simulink model "Heating_room_quick"  (R2023b)
settings: Solver=VariableStepAuto  StartTime=0.0  StopTime=7000  RelTol=1e-3
libraries: fl_lib x21, SimscapeFluids_lib x4, nesl_utility x3
settings Model: Creator=Fahim  LastModifiedBy=Tanzi
settings SimscapeCC: SimscapeLogType=all

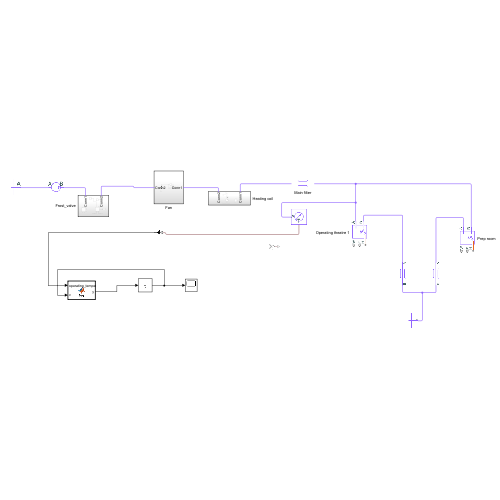
[thumbnail: Simulink's stored preview of the top-level diagram]
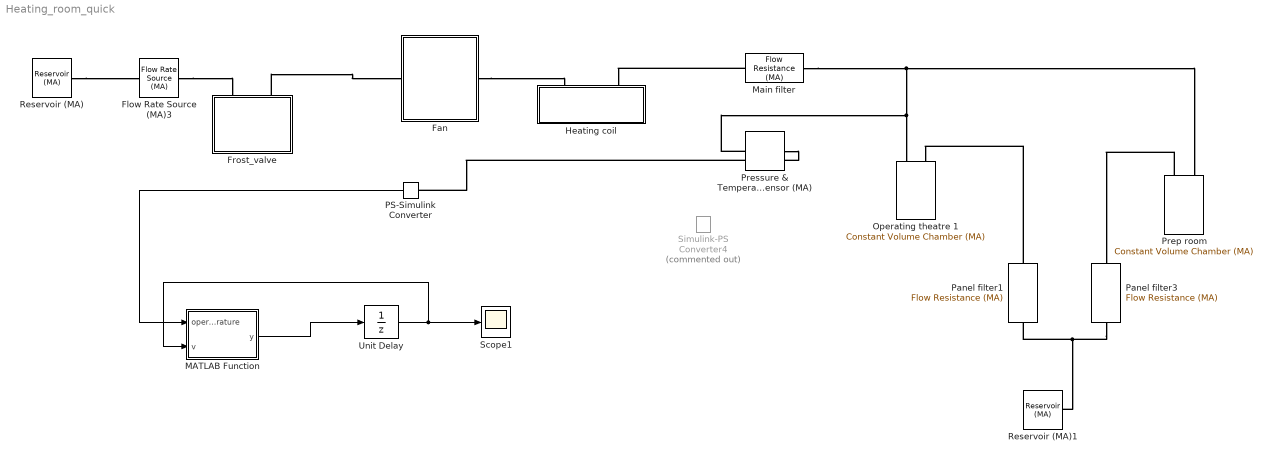
== system Heating_room_quick ==
  Fan : Subsystem
  Flow Rate Source (MA)3 : fl_lib/Moist Air/Sources/Flow Rate Source (MA)  source_type=foundation.enum.constant_controlled.constant  flow_type=foundation.enum.mass_volumetric_flow.mass  mass_flow=1.2 kg/s  volumetric_flow=1 m^3/s  volumetric_flow_conditions=foundation.enum.volumetric_flow_conditions.actual  p_std=0.101325 MPa  T_std=20 degC  RH_std=0.65  power_spec=foundation.enum.power_spec.none  area_A=1.2 m^2  area_B=1.2 m^2
      settings: InternalSimscapePortConfiguration="{\"Bottom\":[],\"Left\":[{\"id\":\"A\",\"label\":\"A\",\"type\":\"foundation.moist_air.moist_air\"}],\"Right\":[{\"id\":\"B\",\"label\":\"B\",\"type\":\"foundation.moist_air.moist_air\"}],\"Top\":[]}"
  Frost_valve : Subsystem
  Heating coil : Subsystem
  MATLAB Function : MATLAB Function  TreatAsAtomicUnit=on
  Main filter : fl_lib/Moist Air/Elements/Flow Resistance (MA)  delta_p_nominal=0.001 MPa  mdot_nominal=2.7 kg/s  rho_nominal=1.2 kg/m^3  area=1.2 m^2  laminar_fraction=1e-3
  Operating theatre 1 : fl_lib/Moist Air/Elements/Constant Volume Chamber (MA)  volume=157 m^3  num_ports=foundation.enum.num_ports.two  area_A=1.2 m^2  area_B=1.2 m^2  area_C=1.2 m^2  area_D=0.01 m^2  RH_ws=1  time_constant=1e-3 s  moisture_trace_gas_source=foundation.enum.moisture_trace_gas_source.none  moisture_source_spec=foundation.enum.moisture_source_spec.vapor  moisture_mass_flow=0 kg/s  moisture_temperature_spec=foundation.enum.temperature_spec.atmospheric  moisture_temperature=293.15 K  trace_gas_mass_flow=0 kg/s  trace_gas_temperature_spec=foundation.enum.temperature_spec.atmospheric  trace_gas_temperature=293.15 K  p_I_specify=off  p_I_priority=High  p_I=0.101325 MPa  p_I_nominal_specify=off  p_I_nominal_unit=MPa  p_I_nominal_value=1  T_I_specify=off  T_I_priority=High  T_I=293.15 K  T_I_nominal_specify=off  T_I_nominal_unit=K  T_I_nominal_value=1  RH_I_specify=off  RH_I_priority=High  RH_I=0  RH_I_nominal_specify=off  RH_I_nominal_unit=1  RH_I_nominal_value=1  x_w_I_specify=off  x_w_I_priority=None  x_w_I=0  x_w_I_nominal_specify=off  x_w_I_nominal_unit=1  x_w_I_nominal_value=1  y_w_I_specify=off  y_w_I_priority=None  y_w_I=0  y_w_I_nominal_specify=off  y_w_I_nominal_unit=1  y_w_I_nominal_value=1  HR_I_specify=off  HR_I_priority=None  HR_I=0  HR_I_nominal_specify=off  HR_I_nominal_unit=1  HR_I_nominal_value=1  x_g_I_specify=off  x_g_I_priority=High  x_g_I=0  x_g_I_nominal_specify=off  x_g_I_nominal_unit=1  x_g_I_nominal_value=1  y_g_I_specify=off  y_g_I_priority=None  y_g_I=0  y_g_I_nominal_specify=off  y_g_I_nominal_unit=1  y_g_I_nominal_value=1
      settings: InternalSimscapePortConfiguration="{\"Bottom\":[],\"Left\":[{\"id\":\"A\",\"label\":\"A\",\"type\":\"foundation.moist_air.moist_air\"},{\"id\":\"B\",\"label\":\"B\",\"type\":\"foundation.moist_air.moist_air\"}],\"Right\":[{\"id\":\"W\",\"label\":\"W\",\"type\":\"output\"},{\"id\":\"F\",\"label\":\"F\",\"type\":\"output\"},{\"id\":\"H\",\"label\":\"H\",\"type\":\"foundation.thermal.thermal\"}],\"Top\":[]}"
  PS-Simulink Converter : nesl_utility/PS-Simulink Converter  PhysicalDomain=network_engine_domain  SubClassName=ps_output  LeftPortType=input  RightPortType=output  PseudoPeriodic=off  Frequencies=[]  VectorFormat=inherit  Unit=inherit  AffineConversion=off
  Panel filter1 : fl_lib/Moist Air/Elements/Flow Resistance (MA)  delta_p_nominal=0.001 MPa  mdot_nominal=0.1 kg/s  rho_nominal=0 kg/m^3  area=0.01 m^2  laminar_fraction=1e-3
  Panel filter3 : fl_lib/Moist Air/Elements/Flow Resistance (MA)  delta_p_nominal=0.001 MPa  mdot_nominal=0.1 kg/s  rho_nominal=0 kg/m^3  area=0.01 m^2  laminar_fraction=1e-3
  Prep room : fl_lib/Moist Air/Elements/Constant Volume Chamber (MA)  volume=157 m^3  num_ports=foundation.enum.num_ports.two  area_A=1.2 m^2  area_B=1.2 m^2  area_C=1.2 m^2  area_D=0.01 m^2  RH_ws=1  time_constant=1e-3 s  moisture_trace_gas_source=foundation.enum.moisture_trace_gas_source.none  moisture_source_spec=foundation.enum.moisture_source_spec.vapor  moisture_mass_flow=0 kg/s  moisture_temperature_spec=foundation.enum.temperature_spec.atmospheric  moisture_temperature=293.15 K  trace_gas_mass_flow=0 kg/s  trace_gas_temperature_spec=foundation.enum.temperature_spec.atmospheric  trace_gas_temperature=293.15 K  p_I_specify=off  p_I_priority=High  p_I=0.101325 MPa  p_I_nominal_specify=off  p_I_nominal_unit=MPa  p_I_nominal_value=1  T_I_specify=off  T_I_priority=High  T_I=293.15 K  T_I_nominal_specify=off  T_I_nominal_unit=K  T_I_nominal_value=1  RH_I_specify=off  RH_I_priority=High  RH_I=0  RH_I_nominal_specify=off  RH_I_nominal_unit=1  RH_I_nominal_value=1  x_w_I_specify=off  x_w_I_priority=None  x_w_I=0  x_w_I_nominal_specify=off  x_w_I_nominal_unit=1  x_w_I_nominal_value=1  y_w_I_specify=off  y_w_I_priority=None  y_w_I=0  y_w_I_nominal_specify=off  y_w_I_nominal_unit=1  y_w_I_nominal_value=1  HR_I_specify=off  HR_I_priority=None  HR_I=0  HR_I_nominal_specify=off  HR_I_nominal_unit=1  HR_I_nominal_value=1  x_g_I_specify=off  x_g_I_priority=High  x_g_I=0  x_g_I_nominal_specify=off  x_g_I_nominal_unit=1  x_g_I_nominal_value=1  y_g_I_specify=off  y_g_I_priority=None  y_g_I=0  y_g_I_nominal_specify=off  y_g_I_nominal_unit=1  y_g_I_nominal_value=1
      settings: InternalSimscapePortConfiguration="{\"Bottom\":[],\"Left\":[{\"id\":\"A\",\"label\":\"A\",\"type\":\"foundation.moist_air.moist_air\"},{\"id\":\"B\",\"label\":\"B\",\"type\":\"foundation.moist_air.moist_air\"}],\"Right\":[{\"id\":\"W\",\"label\":\"W\",\"type\":\"output\"},{\"id\":\"F\",\"label\":\"F\",\"type\":\"output\"},{\"id\":\"H\",\"label\":\"H\",\"type\":\"foundation.thermal.thermal\"}],\"Top\":[]}"
  Pressure & Temperature Sensor (MA) : fl_lib/Moist Air/Sensors/Pressure & Temperature Sensor (MA)  reference=foundation.enum.MeasurementReference.absolute  pressure=false  pressure_spec=foundation.enum.PressureMeasementSpec.Absolute  temperature=true
      settings: InternalSimscapePortConfiguration="{\"Bottom\":[{\"id\":\"T\",\"label\":\"T\",\"type\":\"output\"}],\"Left\":[{\"id\":\"A\",\"label\":\"A\",\"type\":\"foundation.moist_air.moist_air\"}],\"Right\":[],\"Top\":[]}"
  Reservoir (MA) : fl_lib/Moist Air/Elements/Reservoir (MA)  pressure_spec=foundation.enum.pressure_spec.atmospheric  reservoir_pressure=0.101325 MPa  temperature_spec=foundation.enum.temperature_spec.specified  reservoir_temperature=8 degC  moisture_spec=foundation.enum.moistureSpec.RelativeHumidity  reservoir_RH=0.5  reservoir_x_w=0.01  reservoir_y_w=0.01  reservoir_HR=0.01  reservoir_Tw=287 K  trace_gas_spec=foundation.enum.trace_gas_spec.mass_fraction  reservoir_x_g=0.001  reservoir_y_g=0.001  RH_ws=1  area_A=1.2 m^2
  Reservoir (MA)1 : fl_lib/Moist Air/Elements/Reservoir (MA)  pressure_spec=foundation.enum.pressure_spec.atmospheric  reservoir_pressure=0.101325 MPa  temperature_spec=foundation.enum.temperature_spec.specified  reservoir_temperature=18.5 degC  moisture_spec=foundation.enum.moistureSpec.RelativeHumidity  reservoir_RH=0.5  reservoir_x_w=0.01  reservoir_y_w=0.01  reservoir_HR=0.01  reservoir_Tw=287 K  trace_gas_spec=foundation.enum.trace_gas_spec.mass_fraction  reservoir_x_g=0.001  reservoir_y_g=0.001  RH_ws=1  area_A=1.2 m^2
  Scope1 : Scope
  Simulink-PS Converter4 : nesl_utility/Simulink-PS Converter  Commented=on  PhysicalDomain=network_engine_domain  SubClassName=ps_input  LeftPortType=input  RightPortType=output  PseudoPeriodic=off  Frequencies=[]  NoiseDistribution=none  NoiseParameters=[]  Unit=1  AffineConversion=off  FilteringAndDerivatives=provide  SimscapeFilterOrder=1  InputFilterTimeConstant=0.001  UdotUserProvided=0
  Unit Delay : UnitDelay  InitialCondition=8+273  SampleTime=-1  StateName=current_temp  HasFrameUpgradeWarning=on
  wires:
  PS-Simulink Converter/1 -> MATLAB Function/1(operating_temperature)
  MATLAB Function/1(y) -> Unit Delay/1
  Unit Delay/1 -> MATLAB Function/2(v), Scope1/1
  connections:
  Reservoir (MA)/LConn1 -- Flow Rate Source (MA)3/LConn1
  Flow Rate Source (MA)3/RConn1 -- Frost_valve/RConn1
  Frost_valve/RConn2 -- Fan/LConn1
  Fan/RConn1 -- Heating coil/RConn1
  Main filter/LConn1 -- Heating coil/RConn2
  Panel filter3/RConn1 -- Panel filter1/RConn1 -- Reservoir (MA)1/LConn1
  Prep room/LConn1 -- Panel filter3/LConn1
  Panel filter1/LConn1 -- Operating theatre 1/LConn2
  Main filter/RConn1 -- Pressure & Temperature Sensor (MA)/LConn1 -- Operating theatre 1/LConn1 -- Prep room/LConn2
  Pressure & Temperature Sensor (MA)/RConn1 -- PS-Simulink Converter/LConn1

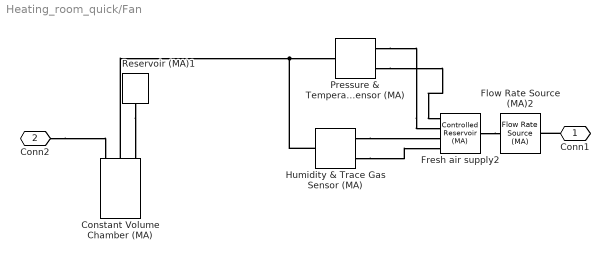
== system Heating_room_quick/Fan ==
  Constant Volume Chamber (MA) : fl_lib/Moist Air/Elements/Constant Volume Chamber (MA)  volume=3.6 m^3  num_ports=foundation.enum.num_ports.three  area_A=1.2 m^2  area_B=1.2 m^2  area_C=1.2 m^2  area_D=0.01 m^2  RH_ws=1  time_constant=1e-3 s  moisture_trace_gas_source=foundation.enum.moisture_trace_gas_source.none  moisture_source_spec=foundation.enum.moisture_source_spec.vapor  moisture_mass_flow=0 kg/s  moisture_temperature_spec=foundation.enum.temperature_spec.atmospheric  moisture_temperature=293.15 K  trace_gas_mass_flow=0 kg/s  trace_gas_temperature_spec=foundation.enum.temperature_spec.atmospheric  trace_gas_temperature=293.15 K  p_I_specify=off  p_I_priority=High  p_I=0.101325 MPa  p_I_nominal_specify=off  p_I_nominal_unit=MPa  p_I_nominal_value=1  T_I_specify=off  T_I_priority=High  T_I=293.15 K  T_I_nominal_specify=off  T_I_nominal_unit=K  T_I_nominal_value=1  RH_I_specify=off  RH_I_priority=High  RH_I=0  RH_I_nominal_specify=off  RH_I_nominal_unit=1  RH_I_nominal_value=1  x_w_I_specify=off  x_w_I_priority=None  x_w_I=0  x_w_I_nominal_specify=off  x_w_I_nominal_unit=1  x_w_I_nominal_value=1  y_w_I_specify=off  y_w_I_priority=None  y_w_I=0  y_w_I_nominal_specify=off  y_w_I_nominal_unit=1  y_w_I_nominal_value=1  HR_I_specify=off  HR_I_priority=None  HR_I=0  HR_I_nominal_specify=off  HR_I_nominal_unit=1  HR_I_nominal_value=1  x_g_I_specify=off  x_g_I_priority=High  x_g_I=0  x_g_I_nominal_specify=off  x_g_I_nominal_unit=1  x_g_I_nominal_value=1  y_g_I_specify=off  y_g_I_priority=None  y_g_I=0  y_g_I_nominal_specify=off  y_g_I_nominal_unit=1  y_g_I_nominal_value=1
      settings: InternalSimscapePortConfiguration="{\"Bottom\":[],\"Left\":[{\"id\":\"A\",\"label\":\"A\",\"type\":\"foundation.moist_air.moist_air\"},{\"id\":\"B\",\"label\":\"B\",\"type\":\"foundation.moist_air.moist_air\"},{\"id\":\"C\",\"label\":\"C\",\"type\":\"foundation.moist_air.moist_air\"}],\"Right\":[{\"id\":\"W\",\"label\":\"W\",\"type\":\"output\"},{\"id\":\"F\",\"label\":\"F\",\"type\":\"output\"},{\"id\":\"H\",\"label\":\"H\",\"type\":\"foundation.thermal.thermal\"}],\"Top\":[]}"
  Flow Rate Source (MA)2 : fl_lib/Moist Air/Sources/Flow Rate Source (MA)  source_type=foundation.enum.constant_controlled.constant  flow_type=foundation.enum.mass_volumetric_flow.mass  mass_flow=2.7 kg/s  volumetric_flow=1 m^3/s  volumetric_flow_conditions=foundation.enum.volumetric_flow_conditions.actual  p_std=0.101325 MPa  T_std=20 degC  RH_std=0.65  power_spec=foundation.enum.power_spec.none  area_A=1.2 m^2  area_B=1.2 m^2
      settings: InternalSimscapePortConfiguration="{\"Bottom\":[],\"Left\":[{\"id\":\"A\",\"label\":\"A\",\"type\":\"foundation.moist_air.moist_air\"}],\"Right\":[{\"id\":\"B\",\"label\":\"B\",\"type\":\"foundation.moist_air.moist_air\"}],\"Top\":[]}"
  Fresh air supply2 : fl_lib/Moist Air/Elements/Controlled Reservoir (MA)  moisture_spec=foundation.enum.moistureSpec.RelativeHumidity  trace_gas_spec=foundation.enum.trace_gas_spec.mass_fraction  RH_ws=1  area_A=1.2 m^2  input_error_spec=foundation.enum.input_range_error.error
      settings: InternalSimscapePortConfiguration="{\"Bottom\":[],\"Left\":[{\"id\":\"A\",\"label\":\"A\",\"type\":\"foundation.moist_air.moist_air\"}],\"Right\":[{\"id\":\"T\",\"label\":\"T\",\"type\":\"input\"},{\"id\":\"P\",\"label\":\"P\",\"type\":\"input\"},{\"id\":\"W\",\"label\":\"W\",\"type\":\"input\"},{\"id\":\"G\",\"label\":\"G\",\"type\":\"input\"}],\"Top\":[]}"
  Humidity & Trace Gas Sensor (MA) : fl_lib/Moist Air/Sensors/Humidity & Trace Gas Sensor (MA)  moisture_on=true  moisture_spec=foundation.enum.moistureSpec.RelativeHumidity  trace_gas_on=true  trace_gas_spec=foundation.enum.trace_gas_spec.mass_fraction
      settings: InternalSimscapePortConfiguration="{\"Bottom\":[],\"Left\":[{\"id\":\"A\",\"label\":\"A\",\"type\":\"foundation.moist_air.moist_air\"}],\"Right\":[{\"id\":\"W\",\"label\":\"W\",\"type\":\"output\"},{\"id\":\"G\",\"label\":\"G\",\"type\":\"output\"}],\"Top\":[]}"
  Pressure & Temperature Sensor (MA) : fl_lib/Moist Air/Sensors/Pressure & Temperature Sensor (MA)  reference=foundation.enum.MeasurementReference.absolute  pressure=true  pressure_spec=foundation.enum.PressureMeasementSpec.Absolute  temperature=true
      settings: InternalSimscapePortConfiguration="{\"Bottom\":[{\"id\":\"T\",\"label\":\"T\",\"type\":\"output\"}],\"Left\":[{\"id\":\"A\",\"label\":\"A\",\"type\":\"foundation.moist_air.moist_air\"}],\"Right\":[{\"id\":\"Pa\",\"label\":\"Pa\",\"type\":\"output\"}],\"Top\":[]}"
  Reservoir (MA)1 : fl_lib/Moist Air/Elements/Reservoir (MA)  pressure_spec=foundation.enum.pressure_spec.atmospheric  reservoir_pressure=0.101325 MPa  temperature_spec=foundation.enum.temperature_spec.specified  reservoir_temperature=20 degC  moisture_spec=foundation.enum.moistureSpec.RelativeHumidity  reservoir_RH=0.5  reservoir_x_w=0.01  reservoir_y_w=0.01  reservoir_HR=0.01  reservoir_Tw=287 K  trace_gas_spec=foundation.enum.trace_gas_spec.mass_fraction  reservoir_x_g=0.001  reservoir_y_g=0.001  RH_ws=1  area_A=1.2 m^2
  Conn1 : PMIOPort  Side=Right
  Conn2 : PMIOPort  Port=2  Side=Left
  connections:
  Humidity & Trace Gas Sensor (MA)/RConn2 -- Fresh air supply2/RConn4
  Pressure & Temperature Sensor (MA)/RConn2 -- Fresh air supply2/RConn1
  Fresh air supply2/LConn1 -- Flow Rate Source (MA)2/LConn1
  Conn1/RConn1 -- Flow Rate Source (MA)2/RConn1
  Reservoir (MA)1/LConn1 -- Constant Volume Chamber (MA)/LConn3
  Humidity & Trace Gas Sensor (MA)/LConn1 -- Constant Volume Chamber (MA)/LConn2 -- Pressure & Temperature Sensor (MA)/LConn1
  Pressure & Temperature Sensor (MA)/RConn1 -- Fresh air supply2/RConn2
  Humidity & Trace Gas Sensor (MA)/RConn1 -- Fresh air supply2/RConn3
  Conn2/RConn1 -- Constant Volume Chamber (MA)/LConn1

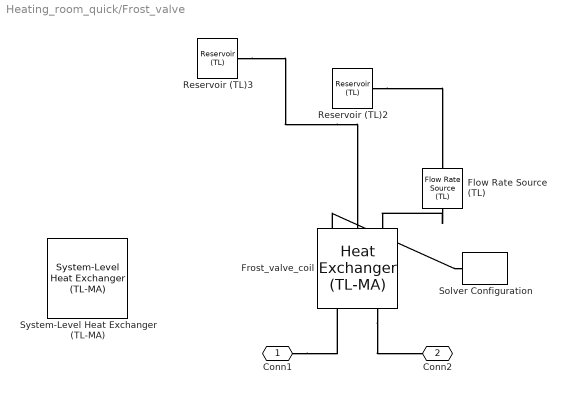
== system Heating_room_quick/Frost_valve ==
  Flow Rate Source (TL) : fl_lib/Thermal Liquid/Sources/Flow Rate Source (TL)  source_type=foundation.enum.constant_controlled.constant  flow_type=foundation.enum.mass_volumetric_flow.mass  mass_flow=0.31 kg/s  volumetric_flow=0 m^3/s  power_spec=foundation.enum.power_spec.none  area=0.44 in^2
      settings: InternalSimscapePortConfiguration="{\"Bottom\":[],\"Left\":[{\"id\":\"A\",\"label\":\"A\",\"type\":\"foundation.thermal_liquid.thermal_liquid\"}],\"Right\":[{\"id\":\"B\",\"label\":\"B\",\"type\":\"foundation.thermal_liquid.thermal_liquid\"}],\"Top\":[]}"
  Frost_valve_coil : SimscapeFluids_lib/Fluid Network Interfaces/Heat Exchangers/Heat Exchanger (TL-MA)  flow_arrangement=fluids.interfaces.heat_exchangers.enum.FlowArrangementTLMA.Cross  cross_flow_arrangement=fluids.interfaces.heat_exchangers.enum.CrossFlowArrangementTLMA.UnmixedUnmixed  R_wall=0 K/kW  area_A1=0.44 in^2  area_B1=0.44 in^2  area_A2=1.2 m^2  area_B2=1.2 m^2  flow_geometry_TL=fluids.interfaces.heat_exchangers.enum.FlowGeometryTL.InsideTubes  tube_num_TL=14  tube_length_TL=1.2 m  tube_cross_section_TL=fluids.interfaces.heat_exchangers.enum.TubeCrossSection.Circular  tube_diameter_TL=0.55 in  tube_width_TL=0.05 m  tube_height_TL=0.05 m  tube_inner_diameter_TL=0.05 m  tube_outer_diameter_TL=0.1 m  tube_flow_area_TL=0.002 m^2  tube_wetted_perimeter_TL=0.15 m  tube_heat_perimeter_TL=0.15 m  tube_pressure_loss_spec_TL=fluids.interfaces.heat_exchangers.enum.TubePressureLossSpec.Haaland  tube_loss_coeff_TL=10  tube_local_pressure_loss_spec_TL=fluids.thermal_liquid.pipes_fittings.enum.LocalLossSpec.AggregateLength  tube_length_add_TL=0.024 in  tube_local_loss_coefficient_TL=0.1  tube_roughness_pressure_TL=15e-6 m  tube_Re_lam_pressure_TL=2000  tube_Re_tur_pressure_TL=4000  tube_shape_factor_generic_TL=64  tube_heat_coeff_spec_TL=fluids.interfaces.heat_exchangers.enum.TubeHeatCoeffSpec.Gneilinski  tube_colburn_coeff_TL=[.023, .8, .33]  tube_roughness_heat_TL=15e-6 m  tube_Re_lam_heat_TL=2000  tube_Re_tur_heat_TL=4000  tube_Nu_lam_generic_TL=3.66  bank_arrangement_TL=fluids.interfaces.heat_exchangers.enum.BankArrangement.Inline  bank_num_rows_TL=5  bank_tubes_per_row_TL=5  bank_width_TL=1 m  bank_tube_diameter_TL=0.05 m  bank_longitudinal_pitch_TL=0.15 m  bank_transverse_pitch_TL=0.15 m  bank_pressure_loss_spec_TL=fluids.interfaces.heat_exchangers.enum.BankPressureLossSpec.Martin  bank_euler_TL=10  bank_heat_coeff_spec_TL=fluids.interfaces.heat_exchangers.enum.BankHeatCoeffSpec.Martin  bank_colburn_coeff_TL=[.27, .63, .36]  generic_flow_area_TL=0.01 m^2  generic_heat_area_TL=2 m^2  generic_volume_TL=0.05 m^3  generic_loss_coeff_TL=10  generic_colburn_coeff_TL=[.023, .8, .33]  fouling_factor_TL=0 K*m^2/kW  fin_area_TL=0 mm^2  fin_efficiency_TL=0.5  p_init_TL=1 bar  T_init_TL=99 degC  flow_geometry_MA=fluids.interfaces.heat_exchangers.enum.FlowGeometryMA.AcrossTubeBank  tube_num_MA=25  tube_length_MA=1 m  tube_cross_section_MA=fluids.interfaces.heat_exchangers.enum.TubeCrossSection.Circular  tube_diameter_MA=0.05 m  tube_width_MA=0.05 m  tube_height_MA=0.05 m  tube_inner_diameter_MA=0.05 m  tube_outer_diameter_MA=0.1 m  tube_flow_area_MA=0.002 m^2  tube_wetted_perimeter_MA=0.15 m  tube_heat_perimeter_MA=0.15 m  tube_pressure_loss_spec_MA=fluids.interfaces.heat_exchangers.enum.TubePressureLossSpec.Haaland  tube_loss_coeff_MA=10  tube_local_pressure_loss_spec_MA=fluids.moist_air.pipes_fittings.enum.LocalLossSpec.AggregateLength  tube_length_add_MA=0.1 m  tube_local_loss_coefficient_MA=0.1  tube_roughness_pressure_MA=15e-6 m  tube_Re_lam_pressure_MA=2000  tube_Re_tur_pressure_MA=4000  tube_shape_factor_generic_MA=64  tube_heat_coeff_spec_MA=fluids.interfaces.heat_exchangers.enum.TubeHeatCoeffSpec.Gneilinski  tube_colburn_coeff_MA=[.023, .8, .33]  tube_roughness_heat_MA=15e-6 m  tube_Re_lam_heat_MA=2000  tube_Re_tur_heat_MA=4000  tube_Nu_lam_generic_MA=3.66  bank_arrangement_MA=fluids.interfaces.heat_exchangers.enum.BankArrangement.Inline  bank_num_rows_MA=1  bank_tubes_per_row_MA=14  bank_width_MA=1.2 m  bank_tube_diameter_MA=0.65 in  bank_longitudinal_pitch_MA=1.1 in  bank_transverse_pitch_MA=1.1 in  bank_pressure_loss_spec_MA=fluids.interfaces.heat_exchangers.enum.BankPressureLossSpec.Martin  bank_euler_MA=10  bank_heat_coeff_spec_MA=fluids.interfaces.heat_exchangers.enum.BankHeatCoeffSpec.Martin  bank_colburn_coeff_MA=[.27, .63, .36]  generic_flow_area_MA=288 in^2  generic_heat_area_MA=0.0511 m^2  generic_volume_MA=1728 in^3  generic_loss_coeff_MA=10  generic_colburn_coeff_MA=[.023, .8, .33]  fouling_factor_MA=0.1 K*m^2/kW  fin_area_MA=2000 in^2  fin_efficiency_MA=0.6  p_init_MA=1 atm  T_init_MA=14 degC  moisture_spec_MA=foundation.enum.moisture_spec.relative_humidity  RH_init_MA=0.8  x_w_init_MA=0.01  y_w_init_MA=0.01  HR_init_MA=0.01  trace_gas_spec_MA=foundation.enum.trace_gas_spec.mass_fraction  x_g_init_MA=0.001  y_g_init_MA=0.001  RH_ws_MA=1
      settings: InternalSimscapePortConfiguration="{\"Bottom\":[],\"Left\":[{\"id\":\"A1\",\"label\":\"A1\",\"type\":\"foundation.thermal_liquid.thermal_liquid\"},{\"id\":\"B1\",\"label\":\"B1\",\"type\":\"foundation.thermal_liquid.thermal_liquid\"}],\"Right\":[{\"id\":\"A2\",\"label\":\"A2\",\"type\":\"foundation.moist_air.moist_air\"},{\"id\":\"B2\",\"label\":\"B2\",\"type\":\"foundation.moist_air.moist_air\"}],\"Top\":[{\"id\":\"W\",\"label\":\"W\",\"type\":\"output\"}]}"
  Reservoir (TL)2 : fl_lib/Thermal Liquid/Elements/Reservoir (TL)  pressure_spec=foundation.enum.pressure_spec.specified  reservoir_pressure=1 bar  reservoir_temperature=99 degC  area=0.44 in^2
  Reservoir (TL)3 : fl_lib/Thermal Liquid/Elements/Reservoir (TL)  pressure_spec=foundation.enum.pressure_spec.specified  reservoir_pressure=1 bar  reservoir_temperature=89 degC  area=0.44 in^2
  Solver Configuration : nesl_utility/Solver Configuration  PhysicalDomain=network_engine_domain  SubClassName=solver  LeftPortType=input  RightPortType=generic  Tones=[]  Harmonics=[]  SimulateNoise=off  Profile=off  UseLocalSampling=off  EnableSwitchedLinearOptims=on  FrequencyDomain=off  UseCCode=off  RelTol=0.001  AbsTol=0.001  MinStep=1e-09  ToWorkspace=off  RevertToSquareIcSolve=off  NumHomotopyIterations=100  PhasorMode=off  PhasorModeNumHarmonics=1  ConsistencySolver=NEWTON_XTOL_AFTER_FTOL  IndexReductionMethod=DerivativeReplacement  DoDC=off  ResidualTolerance=1e-09  ConsistencyTolSource=GLOBAL  ConsistencyAbsTol=0.001  ConsistencyRelTol=0.001  ConsistencyTolFactor=0.001  UseLocalSolver=off  LocalSolverChoice=NE_BACKWARD_EULER_ADVANCER  ResolveIndetEquations=on  FunctionEvalNumThread=1  LocalSolverSampleTime=0.001  DoFixedCost=off  MaxNonlinIter=3  MaxModeIter=2  ComputeImpulses=off  ImpulseIterations=2  LinearAlgebra=auto  LinearAlgebraNumThread=0  EquationFormulation=NE_TIME_EF  DelaysMemoryBudget=1024  AutomaticFiltering=on  FilteringTimeConstant=0.001  PartitionStorageMethod=AS_NEEDED  PartitionMemoryBudget=1024  PartitionMethod=ROBUST  MultibodyUseLocalSolver=off  MultibodyLocalSolverChoice=ODE1  MultibodyLocalSolverSampleTime=0.001
  System-Level Heat Exchanger (TL-MA) : SimscapeFluids_lib/Fluid Network Interfaces/Heat Exchangers/System-Level Heat Exchanger (TL-MA)  flow_arrangement=fluids.interfaces.heat_exchangers.enum.SystemLevelFlowArrangementTLMA.Cross  wall_thermal_mass=false  mass_wall=1 kg  cp_wall=490 J/(K*kg)  nominal_init_wall=true  T_wall_init=293.15 K  area_A1=0.44 in^2  area_B1=0.44 in^2  area_A2=1.2 m^2  area_B2=1.2 m^2  operating_condition_TL=fluids.interfaces.heat_exchangers.enum.SystemLevelOperatingConditionTLMA.Cooling  mdot_nominal_TL=0.31 kg/s  delta_p_nominal_TL=8 kPa  p_in_nominal_TL=0.101325 MPa  T_in_nominal_TL=99 degC  capacity_spec_TL=fluids.interfaces.heat_exchangers.enum.SystemLevelCapacitySpec.HeatTransfer  Q_nominal=7 kW  T_out_nominal_TL=69 degC  volume_TL=0.00477 m^3  nominal_init_TL=true  p_init_TL=0.101325 MPa  T_init_TL=293.15 K  mdot_nominal_MA=1.2 kg/s  delta_p_nominal_MA=0.001 MPa  p_in_nominal_MA=0.101325 MPa  T_in_nominal_MA=10 degC  inlet_moisture_spec_MA=foundation.enum.moisture_spec.relative_humidity  RH_in_nominal_MA=0.5  x_w_in_nominal_MA=0.01  y_w_in_nominal_MA=0.01  HR_in_nominal_MA=0.01  inlet_trace_gas_spec_MA=foundation.enum.trace_gas_spec.mass_fraction  x_g_in_nominal_MA=0.001  y_g_in_nominal_MA=0.001  volume_MA=0.8 m^3  nominal_init_MA=true  p_init_MA=0.101325 MPa  T_init_MA=293.15 K  moisture_spec_MA=foundation.enum.moisture_spec.relative_humidity  RH_init_MA=0.5  x_w_init_MA=0.01  y_w_init_MA=0.01  HR_init_MA=0.01  trace_gas_spec_MA=foundation.enum.trace_gas_spec.mass_fraction  x_g_init_MA=0.001  y_g_init_MA=0.001  RH_ws_MA=1  a_TL=0.023  b_TL=0.8  c_TL=0.33  a_MA=0.023  b_MA=0.8  c_MA=0.33
      settings: InternalSimscapePortConfiguration="{\"Bottom\":[],\"Left\":[{\"id\":\"A1\",\"label\":\"A1\",\"type\":\"foundation.thermal_liquid.thermal_liquid\"},{\"id\":\"B1\",\"label\":\"B1\",\"type\":\"foundation.thermal_liquid.thermal_liquid\"}],\"Right\":[{\"id\":\"A2\",\"label\":\"A2\",\"type\":\"foundation.moist_air.moist_air\"},{\"id\":\"B2\",\"label\":\"B2\",\"type\":\"foundation.moist_air.moist_air\"}],\"Top\":[{\"id\":\"Q1\",\"label\":\"Q1\",\"type\":\"output\"},{\"id\":\"Q2\",\"label\":\"Q2\",\"type\":\"output\"},{\"id\":\"W\",\"label\":\"W\",\"type\":\"output\"}]}"
  Conn1 : PMIOPort  Side=Right
  Conn2 : PMIOPort  Port=2  Side=Right
  connections:
  Reservoir (TL)2/LConn1 -- Flow Rate Source (TL)/LConn1
  Flow Rate Source (TL)/RConn1 -- Frost_valve_coil/LConn1
  Reservoir (TL)3/LConn1 -- Frost_valve_coil/LConn2
  Conn1/RConn1 -- Frost_valve_coil/RConn2
  Frost_valve_coil/RConn1 -- Conn2/RConn1
  Frost_valve_coil/LConn3 -- Solver Configuration/RConn1

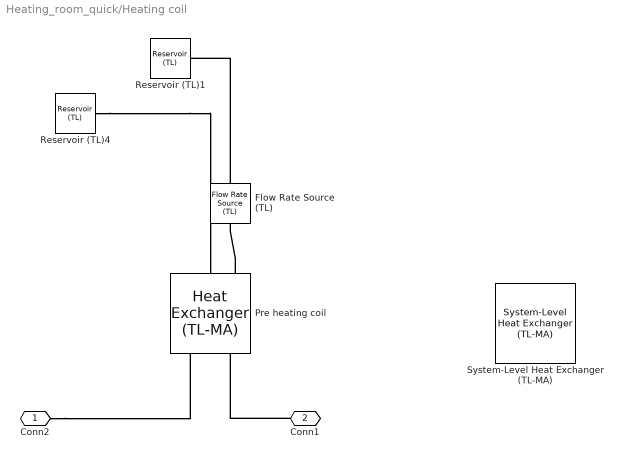
== system Heating_room_quick/Heating coil ==
  Flow Rate Source (TL) : fl_lib/Thermal Liquid/Sources/Flow Rate Source (TL)  source_type=foundation.enum.constant_controlled.constant  flow_type=foundation.enum.mass_volumetric_flow.mass  mass_flow=0.41 kg/s  volumetric_flow=0 m^3/s  power_spec=foundation.enum.power_spec.none  area=0.44 in^2
      settings: InternalSimscapePortConfiguration="{\"Bottom\":[],\"Left\":[{\"id\":\"A\",\"label\":\"A\",\"type\":\"foundation.thermal_liquid.thermal_liquid\"}],\"Right\":[{\"id\":\"B\",\"label\":\"B\",\"type\":\"foundation.thermal_liquid.thermal_liquid\"}],\"Top\":[]}"
  Pre heating coil : SimscapeFluids_lib/Fluid Network Interfaces/Heat Exchangers/Heat Exchanger (TL-MA)  flow_arrangement=fluids.interfaces.heat_exchangers.enum.FlowArrangementTLMA.Cross  cross_flow_arrangement=fluids.interfaces.heat_exchangers.enum.CrossFlowArrangementTLMA.UnmixedUnmixed  R_wall=0 K/kW  area_A1=0.44 in^2  area_B1=0.44 in^2  area_A2=1.2 m^2  area_B2=1.2 m^2  flow_geometry_TL=fluids.interfaces.heat_exchangers.enum.FlowGeometryTL.InsideTubes  tube_num_TL=14  tube_length_TL=1.2 m  tube_cross_section_TL=fluids.interfaces.heat_exchangers.enum.TubeCrossSection.Circular  tube_diameter_TL=0.55 in  tube_width_TL=0.05 m  tube_height_TL=0.05 m  tube_inner_diameter_TL=0.05 m  tube_outer_diameter_TL=0.1 m  tube_flow_area_TL=0.002 m^2  tube_wetted_perimeter_TL=0.15 m  tube_heat_perimeter_TL=0.15 m  tube_pressure_loss_spec_TL=fluids.interfaces.heat_exchangers.enum.TubePressureLossSpec.Haaland  tube_loss_coeff_TL=10  tube_local_pressure_loss_spec_TL=fluids.thermal_liquid.pipes_fittings.enum.LocalLossSpec.AggregateLength  tube_length_add_TL=0.024 in  tube_local_loss_coefficient_TL=0.1  tube_roughness_pressure_TL=15e-6 m  tube_Re_lam_pressure_TL=2000  tube_Re_tur_pressure_TL=4000  tube_shape_factor_generic_TL=64  tube_heat_coeff_spec_TL=fluids.interfaces.heat_exchangers.enum.TubeHeatCoeffSpec.Gneilinski  tube_colburn_coeff_TL=[.023, .8, .33]  tube_roughness_heat_TL=15e-6 m  tube_Re_lam_heat_TL=2000  tube_Re_tur_heat_TL=4000  tube_Nu_lam_generic_TL=3.66  bank_arrangement_TL=fluids.interfaces.heat_exchangers.enum.BankArrangement.Inline  bank_num_rows_TL=5  bank_tubes_per_row_TL=5  bank_width_TL=1 m  bank_tube_diameter_TL=0.05 m  bank_longitudinal_pitch_TL=0.15 m  bank_transverse_pitch_TL=0.15 m  bank_pressure_loss_spec_TL=fluids.interfaces.heat_exchangers.enum.BankPressureLossSpec.Martin  bank_euler_TL=10  bank_heat_coeff_spec_TL=fluids.interfaces.heat_exchangers.enum.BankHeatCoeffSpec.Martin  bank_colburn_coeff_TL=[.27, .63, .36]  generic_flow_area_TL=0.01 m^2  generic_heat_area_TL=2 m^2  generic_volume_TL=0.05 m^3  generic_loss_coeff_TL=10  generic_colburn_coeff_TL=[.023, .8, .33]  fouling_factor_TL=0 K*m^2/kW  fin_area_TL=0 mm^2  fin_efficiency_TL=0.5  p_init_TL=1 bar  T_init_TL=90 degC  flow_geometry_MA=fluids.interfaces.heat_exchangers.enum.FlowGeometryMA.AcrossTubeBank  tube_num_MA=25  tube_length_MA=1 m  tube_cross_section_MA=fluids.interfaces.heat_exchangers.enum.TubeCrossSection.Circular  tube_diameter_MA=0.05 m  tube_width_MA=0.05 m  tube_height_MA=0.05 m  tube_inner_diameter_MA=0.05 m  tube_outer_diameter_MA=0.1 m  tube_flow_area_MA=0.002 m^2  tube_wetted_perimeter_MA=0.15 m  tube_heat_perimeter_MA=0.15 m  tube_pressure_loss_spec_MA=fluids.interfaces.heat_exchangers.enum.TubePressureLossSpec.Haaland  tube_loss_coeff_MA=10  tube_local_pressure_loss_spec_MA=fluids.moist_air.pipes_fittings.enum.LocalLossSpec.AggregateLength  tube_length_add_MA=0.1 m  tube_local_loss_coefficient_MA=0.1  tube_roughness_pressure_MA=15e-6 m  tube_Re_lam_pressure_MA=2000  tube_Re_tur_pressure_MA=4000  tube_shape_factor_generic_MA=64  tube_heat_coeff_spec_MA=fluids.interfaces.heat_exchangers.enum.TubeHeatCoeffSpec.Gneilinski  tube_colburn_coeff_MA=[.023, .8, .33]  tube_roughness_heat_MA=15e-6 m  tube_Re_lam_heat_MA=2000  tube_Re_tur_heat_MA=4000  tube_Nu_lam_generic_MA=3.66  bank_arrangement_MA=fluids.interfaces.heat_exchangers.enum.BankArrangement.Inline  bank_num_rows_MA=1  bank_tubes_per_row_MA=14  bank_width_MA=1.2 m  bank_tube_diameter_MA=0.55 in  bank_longitudinal_pitch_MA=1.1 in  bank_transverse_pitch_MA=1.1 in  bank_pressure_loss_spec_MA=fluids.interfaces.heat_exchangers.enum.BankPressureLossSpec.Martin  bank_euler_MA=10  bank_heat_coeff_spec_MA=fluids.interfaces.heat_exchangers.enum.BankHeatCoeffSpec.Martin  bank_colburn_coeff_MA=[.27, .63, .36]  generic_flow_area_MA=288 in^2  generic_heat_area_MA=0.0511 m^2  generic_volume_MA=1728 in^3  generic_loss_coeff_MA=10  generic_colburn_coeff_MA=[.023, .8, .33]  fouling_factor_MA=0.1 K*m^2/kW  fin_area_MA=1130 in^2  fin_efficiency_MA=0.6  p_init_MA=1 atm  T_init_MA=14 degC  moisture_spec_MA=foundation.enum.moisture_spec.relative_humidity  RH_init_MA=0.8  x_w_init_MA=0.01  y_w_init_MA=0.01  HR_init_MA=0.01  trace_gas_spec_MA=foundation.enum.trace_gas_spec.mass_fraction  x_g_init_MA=0.001  y_g_init_MA=0.001  RH_ws_MA=1
      settings: InternalSimscapePortConfiguration="{\"Bottom\":[],\"Left\":[{\"id\":\"A1\",\"label\":\"A1\",\"type\":\"foundation.thermal_liquid.thermal_liquid\"},{\"id\":\"B1\",\"label\":\"B1\",\"type\":\"foundation.thermal_liquid.thermal_liquid\"}],\"Right\":[{\"id\":\"A2\",\"label\":\"A2\",\"type\":\"foundation.moist_air.moist_air\"},{\"id\":\"B2\",\"label\":\"B2\",\"type\":\"foundation.moist_air.moist_air\"}],\"Top\":[{\"id\":\"W\",\"label\":\"W\",\"type\":\"output\"}]}"
  Reservoir (TL)1 : fl_lib/Thermal Liquid/Elements/Reservoir (TL)  pressure_spec=foundation.enum.pressure_spec.specified  reservoir_pressure=1 bar  reservoir_temperature=90 degC  area=0.44 in^2
  Reservoir (TL)4 : fl_lib/Thermal Liquid/Elements/Reservoir (TL)  pressure_spec=foundation.enum.pressure_spec.specified  reservoir_pressure=1 bar  reservoir_temperature=90 degC  area=0.44 in^2
  System-Level Heat Exchanger (TL-MA) : SimscapeFluids_lib/Fluid Network Interfaces/Heat Exchangers/System-Level Heat Exchanger (TL-MA)  flow_arrangement=fluids.interfaces.heat_exchangers.enum.SystemLevelFlowArrangementTLMA.Cross  wall_thermal_mass=false  mass_wall=1 kg  cp_wall=490 J/(K*kg)  nominal_init_wall=true  T_wall_init=293.15 K  area_A1=0.44 in^2  area_B1=0.44 in^2  area_A2=1.2 m^2  area_B2=1.2 m^2  operating_condition_TL=fluids.interfaces.heat_exchangers.enum.SystemLevelOperatingConditionTLMA.Cooling  mdot_nominal_TL=0.31 kg/s  delta_p_nominal_TL=8 kPa  p_in_nominal_TL=0.101325 MPa  T_in_nominal_TL=99 degC  capacity_spec_TL=fluids.interfaces.heat_exchangers.enum.SystemLevelCapacitySpec.HeatTransfer  Q_nominal=7 kW  T_out_nominal_TL=69 degC  volume_TL=0.00477 m^3  nominal_init_TL=true  p_init_TL=0.101325 MPa  T_init_TL=293.15 K  mdot_nominal_MA=1.2 kg/s  delta_p_nominal_MA=0.001 MPa  p_in_nominal_MA=0.101325 MPa  T_in_nominal_MA=10 degC  inlet_moisture_spec_MA=foundation.enum.moisture_spec.relative_humidity  RH_in_nominal_MA=0.5  x_w_in_nominal_MA=0.01  y_w_in_nominal_MA=0.01  HR_in_nominal_MA=0.01  inlet_trace_gas_spec_MA=foundation.enum.trace_gas_spec.mass_fraction  x_g_in_nominal_MA=0.001  y_g_in_nominal_MA=0.001  volume_MA=0.8 m^3  nominal_init_MA=true  p_init_MA=0.101325 MPa  T_init_MA=293.15 K  moisture_spec_MA=foundation.enum.moisture_spec.relative_humidity  RH_init_MA=0.5  x_w_init_MA=0.01  y_w_init_MA=0.01  HR_init_MA=0.01  trace_gas_spec_MA=foundation.enum.trace_gas_spec.mass_fraction  x_g_init_MA=0.001  y_g_init_MA=0.001  RH_ws_MA=1  a_TL=0.023  b_TL=0.8  c_TL=0.33  a_MA=0.023  b_MA=0.8  c_MA=0.33
      settings: InternalSimscapePortConfiguration="{\"Bottom\":[],\"Left\":[{\"id\":\"A1\",\"label\":\"A1\",\"type\":\"foundation.thermal_liquid.thermal_liquid\"},{\"id\":\"B1\",\"label\":\"B1\",\"type\":\"foundation.thermal_liquid.thermal_liquid\"}],\"Right\":[{\"id\":\"A2\",\"label\":\"A2\",\"type\":\"foundation.moist_air.moist_air\"},{\"id\":\"B2\",\"label\":\"B2\",\"type\":\"foundation.moist_air.moist_air\"}],\"Top\":[{\"id\":\"Q1\",\"label\":\"Q1\",\"type\":\"output\"},{\"id\":\"Q2\",\"label\":\"Q2\",\"type\":\"output\"},{\"id\":\"W\",\"label\":\"W\",\"type\":\"output\"}]}"
  Conn2 : PMIOPort  Side=Right
  Conn1 : PMIOPort  Port=2  Side=Right
  connections:
  Flow Rate Source (TL)/LConn1 -- Reservoir (TL)1/LConn1
  Pre heating coil/LConn1 -- Flow Rate Source (TL)/RConn1
  Reservoir (TL)4/LConn1 -- Pre heating coil/LConn2
  Conn2/RConn1 -- Pre heating coil/RConn2
  Conn1/RConn1 -- Pre heating coil/RConn1

== matlab function Heating_room_quick/MATLAB Function ==
  data: operating_temperature input; y output; v input
function y = fcn(operating_temperature, v)
% Given parameters
h = 30000; % Convective heat transfer coefficient (W/m^2 K)
mass_air = 203; % Mass of air in the room (kg)
cp = 1005; % Specific heat capacity of air (J/kg K)
A = 1; % Surface area of the vent (m^2)

    % Calculate heat transfer rate from incoming air to the room
Q_in = h * A * (operating_temperature - v);
    
% Calculate change in room temperature using energy balance equation
dT = Q_in / (mass_air * cp);
    
% Update room temperature
y = v + dT;
